simulink model "ECB"  (R2017a)
settings: Solver=ode4  StartTime=0.0  StopTime=1548.3  FixedStep=0.001  RelTol=1e-3  EnableMultiTasking=on
undefined symbols (not defined in the file or in its folder): magnitude, sgn, sigbuilder_block
libraries: simulink x1
(part 1 of 2)
settings Model: SimulationMode=accelerator  Creator=vepsalj1  LastModifiedBy=jariv
settings OptimizationCC: LifeSpan=inf  AccelVerboseBuild=on
settings DebuggingCC: AlgebraicLoopMsg=none  SFUnexpectedBacktrackingDiag=warning  SFNoUnconditionalDefaultTransitionDiag=warning  SFExecutionAtInitializationDiag=none
settings GRTTargetCC: TargetLangStandard=C89/C90 (ANSI)  GeneratePreprocessorConditionals=Disable all
settings ConfigComp: CovMetricSettings=dw  CovHtmlReporting=on  CovSaveCumulativeToWorkspaceVar=on  CovSaveSingleToWorkspaceVar=on  CovExternalEMLEnable=off

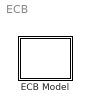
== system ECB ==
  ECB Model : Subsystem  mask{i=4.93, tRout=0.43, m=10500, Jm=0.63, Jt=8, head_wind=0, Cd=0.6, Ad=6.2, fr=0.008, kps=800, kis=0, kds=0, kps_park_multi=10, kpc=0.5, kic=80, kdc=0, Tmax=2080, Tbmax=30000, Rs=55e-3, Ls=5e-4, p=6, flux=0.42, Ppeak=207, Ich=282, Ids=395, soclim=90, vPart=4, aPart=4, x1=192, x2=2, Ah1=45, Rint1=2.5, C1=5, SOC0=85, Ta=20, Tb=20, Nnom=5000, NX=0, Rcor=1, Ccor=1, Ahcor=1, aux=5}
      mask prompts: i "Gear ratio (def 4.93)"; tRout "Tire diameter [m] (def 0.43)"; m "Vehicle mass [kg] (def 10500)"; Jm "Motor inertia [kgm2] (def 0.63)"; Jt "Tire inertia [kgm2] (def 8)"; head_wind "Head wind [m/s] (+ for drag)"; Cd "Coefficient of drag (def 0.493)"; Ad "Vehicle frontal area [m2] (def 6.2)"; fr "Rolling resistance coefficient (def 0.008)"; kps "Speed P gain (def  800)"; kis "Speed I gain (def 0)"; kds "Speed D gain (def 0)"; kps_park_multi "Speed P gain parking multiplier (def 10)"; kpc "Current P gain (def 0.5)"; kic "Current I gain (def 80)"; kdc "Current D gain (def 0)"; Tmax "Max. Motor Torque [Nm] (def 2080)"; Tbmax "Max. Braking Torque [Nm] (def 30 000)"; Rs "Internal resistance [ohm] (def 55e-3)"; Ls "Stator armature inductance [H] (def 5e-4)"; p "Number of pole pairs (def 6)"; flux "Flux induced by magnets [Vs] (def 0.42)"; Ppeak "Motor peak power (kW)"; Ich "Max. motor current when regenerating [A] (def 282)"; Ids "Max. motor current when motoring [A] (def 395)"; soclim "Battery SoC regeneration limit (%) (def 90)"; vPart "Regeneration velocity threshold [km/h] (def 4)"; aPart "Regeneration deceleration threshold [m/s^2] (def 4)"; x1 "Number of modules in series (def 192)"; x2 "Number of modules in parallel  (def 2)"; Ah1 "Nominal cell capacity [Ah] (def 45)"; Rint1 "Internal resistance of a module (mOhm) (@ 20 C) (def 2.5)"; C1 "Capacitance of a module [F] (def 5)"; SOC0 "State-of-Charge (%)"; Ta "Ambient temperature [C] (def 20)"; Tb "Battery temperature (C)"; Nnom "Number of cycles to 80 % aging (def 5000)"; NX "Cycle aging (20 % is EOL, 0 % is new)"; Rcor "Resistance gain"; Ccor "Capacitance gain"; Ahcor "Capacity gain"; aux "Aux power [kW] (constant) (def 5)"
      mask help:
      | Lithium-ion battery
      | - Max. Stepsize 0.2, otherwise there will be vibration in the beginning. Just to be on the safe side, recommended max.step 0.1
      mask init:
      | %MECHANICS
      | Jtot=(Jt*4)+(Jm*i^2);
      | %Four wheel plus the amplified inertia of the motor
      | 
      | %ELECTRONICS
      | PmotPeak=Ppeak*1000;
      | 
      | %BATTERY
      | SOD=[0;2.25000000000000;4;5.75000000000000;7.25000000000000;8.75000000000000;10.2500000000000;11.7500000000000;13.2500000000000;14.7500000000000;16.2500000000000;17.7500000000000;19.2500000000000;20.5000000000000;22;23.5000000000000;25;26.7500000000000;28.2500000000000;29.7500000000000;31.5000000000000;32.7500000000000;34.2500000000000;35.7500000000000;37.2500000000000;39.5000000000000;41.2500000000000;42.7500000000000;44.7500000000000;46.7500000000000;49;51;53.2500000000000;55.5000000000000;57.5000000000000;60;61.7500000000000;64;66.2500000000000;68.2500000000000;70.2500000000000;72.2500000000000;73.7500000000000;75.7500000000000;77.5000000000000;79;80.5000000000000;82;83.5000000000000;84.7500000000000;86.5000000000000;87.7500000000000;89.0000000000000;90.2500000000000;91.5000000000000;92.5000000000000;93.7500000000000;94.5000000000000;95;95.5000000000000;95.7500000000000;96.2500000000000;96.7500000000000;97.0000000000000;97.5000000000000;97.7500000000000;98.2500000000000;98.7500000000000;99.2500000000000;100];
      | VOLT=x1*1.015*[3.30000000000000;3.28450560652396;3.28018348623853;3.27431192660550;3.27308868501529;3.27125382262997;3.27003058103976;3.26819571865443;3.26697247706422;3.26574923547401;3.26452599388379;3.26269113149847;3.26146788990826;3.25963302752294;3.25779816513761;3.25596330275229;3.25474006116208;3.25290519877676;3.25107033639144;3.24862385321101;3.24678899082569;3.24495412844037;3.24311926605505;3.24128440366972;3.23944954128440;3.23761467889908;3.23516819571865;3.23272171253823;3.23027522935780;3.22844036697248;3.22599388379205;3.22354740061162;3.22110091743119;3.21865443425077;3.21559633027523;3.21253822629969;3.20948012232416;3.20703363914373;3.20458715596330;3.20214067278287;3.19969418960245;3.19663608562691;3.19296636085627;3.18868501529052;3.18379204892966;3.17828746177370;3.17278287461774;3.16666666666667;3.15932721712538;3.15076452599388;3.14097859327217;3.12996941896024;3.11712538226300;3.10305810397554;3.08654434250765;3.06880733944954;3.04740061162080;3.02354740061162;2.99785932721713;2.96850152905199;2.93486238532110;2.90061162079511;2.86330275229358;2.82354740061162;2.78012232415902;2.73425076452599;2.68409785932722;2.62782874617737;2.57033639143731;2.50305810397554];
      | 
      | VOLT0=interp1(SOD,VOLT,(1-SOC0/100));
      | % x1=number of cells in series
      | % x2=number of cells in parallel
      | 
      | Ah=x2*Ah1*Ahcor;
      | % Battery Characteristics
      | Qr=3600*Ah; %(coulomb) Nominal capacity in coulombs
      | 
      | N0=(Nnom/20)*NX; %From procentages of aging to number of cycles used
      | 
      | %R as a function of temperature, estimated from AMEsim battery (
      | %R = -0.000000063*Temp.^3+0.00000837*Temp.^2-0.000365*Temp+0.0068)
      | 
      | xx=(Rint1*10^-3)-(-0.000000063*20^3+0.00000837*20^2-0.000365*20);
      | Rint01 = -0.000000063*Tb^3+0.00000837*Tb^2-0.000365*Tb+xx;
      | 
      | Rint02=(x1/x2)*Rint01*Rcor;
      | R1=(2/3)*Rint02; %(ohm) (80 mOhm) (from Gao2002)
      | R2=(1/3)*Rint02; %(ohm) (40 mOhm)(from Gao2002)
      | 
      | Rint=(x1/x2)*Rint1*Rcor;
      | R1=(2/3)*Rint*10^-3; %(ohm) (80 mOhm) (from Gao2002)
      | R2=(1/3)*Rint*10^-3; %(ohm) (40 mOhm)(from Gao2002)
      | 
      | C=(x2/x1)*C1*Ccor;
      | 
      | %% Power converter efficiency
      | effeff=[0.148750893284055 0.459249842031262 0.572831006370283 0.661454547983232 0.702208498156483 0.745300650629634 0.774069453976362 0.802659853674854 0.819870547509622 0.839015378399121 0.851690885251339 0.864745206888717 0.872221885739442 0.879785746841656 0.890777178439945 0.900612362220784 0.905502967085794 0.910295193280307 0.914664248246699 0.916878485285563 0.919785184176078 0.917335161630957 0.920803182958674 0.925793859304388 0.930940164285346 0.936011371736695 0.937121595263058 0.938224789713163 0.941344451389100 0.942389340240952 0.941177012682751 0.942161786791917 0.946805761207415 0.951517305236046 0.956748293196982 0.957192859351870 0.957568033841468 0.956993932406603 0.960453080634668 0.958703134363870 0.958935623923192 0.960813757119483 0.960148641511847;0.382275397060378 0.606575062414118 0.724295084817057 0.763980132419977 0.817545815146612 0.836658234149830 0.850970215271699 0.875397571679227 0.885913726171233 0.897254928610336 0.906002057506642 0.916871389404069 0.925337547906322 0.929573292905226 0.935027508565980 0.934625050493851 0.936779709156045 0.942723985190616 0.945792130928845 0.947960897704374 0.947887831754402 0.950483214667466 0.954939155162541 0.957118148696677 0.962878037248519 0.964085567882039 0.964397321556185 0.966237886367941 0.967550686204577 0.967680328255962 0.968676606501984 0.968600791445791 0.969737387096799 0.970540279155023 0.970270355300112 0.969875112094269 0.970623441746216 0.971620597685068 0.971617448427293 0.973436842558703 0.971015950334548 0.972395281399074 0.972934205141957;0.502794468483159 0.704576784417921 0.780838362491516 0.824760271595067 0.855304468102641 0.874935150583253 0.890548161335983 0.898851103061955 0.911650918822123 0.920752385315524 0.923703036993863 0.938568143297259 0.941262344523035 0.939989162335414 0.947986636638787 0.950531267134112 0.950769184100132 0.953829085066537 0.957748210174090 0.952209232414559 0.959470289301486 0.965800711176068 0.969844708849249 0.970236996539206 0.971698393398446 0.973560393258196 0.972950737175279 0.973910716888667 0.975139162066989 0.975625795237705 0.974938242045002 0.974638822762701 0.975375940537886 0.975427862119037 0.975524897155774 0.977970674599018 0.977066843404792 0.976386481426328 0.978639106804244 0.976987258666757 0.976161252344463 0.974368520302056 0.979968848496111;0.590015102662206 0.757167014367670 0.802721182603195 0.855481189976114 0.875361411684403 0.886491064662271 0.907618702305879 0.917954995694953 0.926135352960324 0.929969047596192 0.934643440724457 0.946673327694363 0.949150648490242 0.952206770632412 0.953620700743328 0.958116293968123 0.960471764182804 0.960022428014383 0.964558913144813 0.964469991899858 0.967188838178770 0.973665568292064 0.973500122873302 0.975787459691329 0.976131734155535 0.975934048502296 0.977728917634797 0.975967753974241 0.977497590850481 0.976961490501139 0.976646573311052 0.976948671343312 0.977003373837591 0.977413505209625 0.977241769484167 0.978136863133043 0.983715860412863 0.972440548088471 0.976031098418230 0.976305098289204 0.983815037717926 0.990000000000000 0.980296964680289;0.642469564171041 0.782143695996117 0.834587558867662 0.867036501869607 0.885404521372931 0.900651198797785 0.918346940196575 0.926228607434163 0.933405508111231 0.940077144823606 0.941875513808993 0.949129235726833 0.955031705790567 0.955638703032255 0.959733157663852 0.961256947439685 0.964228704878266 0.965503729478674 0.967427866304563 0.970406018303361 0.975922234217047 0.976479479306018 0.977524713303582 0.978942094461665 0.977781595580544 0.977114802612142 0.975292354675851 0.977565938254442 0.977663963097884 0.970728918766358 0.978509263236759 0.979294318591674 0.978606184812507 0.980455355005113 0.977717973547513 0.977611212207795 0.977488362388515 0.983520834208511 0.978653676557568 0.977797224149179 0.976671295279777 0.982936790637227 0.974693280544320;0.666854189302077 0.796081554018545 0.853459995484673 0.875731344523075 0.894560218167283 0.910024324986280 0.920660243620183 0.936114908254807 0.937377010306665 0.943946530066235 0.947946898995783 0.955373031072732 0.956645495867027 0.961083778718095 0.961007216676884 0.965157442857362 0.965963755148971 0.968049149876401 0.971312101606815 0.975913333987052 0.975359086105523 0.977443627145109 0.977029983816712 0.978751343960785 0.978669311729546 0.980440204724162 0.984357530160600 0.978582708734772 0.979172562917930 0.978804034312948 0.978996524660769 0.978808094694211 0.978747993277991 0.978709803944595 0.984219208058756 0.978066410331978 0.977474370808590 0.976281712836119 0.976850901804032 0.970232997225184 0.990000000000000 0.990000000000000 0.990000000000000;0.693198974002651 0.812744420563275 0.861303411362365 0.888370040041046 0.899912367804584 0.912416422686382 0.927557031051808 0.934602759564506 0.939933212996785 0.947091254831535 0.951201311892576 0.959125411213696 0.959470857340005 0.961454980867527 0.963471596082249 0.965897069441330 0.967443349261464 0.968159753257309 0.972751289105061 0.976432852036816 0.977478975415255 0.978905952575006 0.978862035952765 0.979306529314671 0.979054079435176 0.979228864872502 0.980328291262954 0.979395165978778 0.979009717648825 0.979197157798663 0.979144584572849 0.979687221448110 0.979867607494733 0.978961695988816 0.982870884306758 0.976036523552125 0.970527543739429 0.990000000000000 0.990000000000000 0.990000000000000 0.990000000000000 0.990000000000000 0.990000000000000;0.723442421271799 0.819434992636961 0.866442600856177 0.887397491216575 0.912904261162542 0.915767451704052 0.930373806731795 0.937079106193214 0.942969048836058 0.948839064874878 0.953173425562567 0.957489332249449 0.963566641747761 0.964127874132415 0.964929847641875 0.966679582560640 0.968946853098627 0.970288863581759 0.975665835406012 0.977412335686879 0.979209315237733 0.978604269795064 0.979819900585854 0.979934412452209 0.980296834612691 0.979389810437186 0.979927925307359 0.979821966114863 0.980113197866812 0.978290737811240 0.978777326301659 0.978275795371243 0.977699190470578 0.976771188346836 0.990000000000000 0.990000000000000 0.990000000000000 0.990000000000000 0.990000000000000 0.990000000000000 0.990000000000000 0.990000000000000 0.990000000000000;0.748379721863994 0.841228290700447 0.864645554182945 0.893076811535185 0.909585899362390 0.920963299154172 0.934746905084107 0.941263940245672 0.943727860504373 0.950708651654628 0.954462263097205 0.960285791762753 0.962938135424456 0.963189598051574 0.965424092681620 0.967948124641425 0.968458535243243 0.974314778624769 0.976814364122101 0.979690184628213 0.979635217015122 0.979521508451437 0.979315060652411 0.980151729989435 0.979576323726992 0.979214145569015 0.980432559684310 0.979463877927784 0.978551029380815 0.978916907697418 0.978331589142382 0.978072711203139 0.990000000000000 0.990000000000000 0.990000000000000 0.990000000000000 0.990000000000000 0.990000000000000 0.990000000000000 0.990000000000000 0.990000000000000 0.990000000000000 0.990000000000000;0.739921993857994 0.842186224128038 0.872808349192410 0.897527110792011 0.911584252711211 0.926021034143323 0.931411696811273 0.943432421331771 0.946957435884837 0.952226260338947 0.955612156419591 0.961031292110199 0.963399102509892 0.965628015212985 0.967341907415101 0.968367188392990 0.970371532378770 0.975428592316753 0.978090341015957 0.978778385764394 0.979356164049638 0.979596787238044 0.979910905936328 0.980438856293780 0.979604150440873 0.979929471066156 0.978964026966460 0.979032120167408 0.978326079936520 0.976905872301957 0.990000000000000 0.990000000000000 0.990000000000000 0.990000000000000 0.990000000000000 0.990000000000000 0.990000000000000 0.990000000000000 0.990000000000000 0.990000000000000 0.990000000000000 0.990000000000000 0.990000000000000;0.764782550308260 0.845852311796918 0.877247852208968 0.900372955117317 0.916038722932507 0.928163498727814 0.936820012399945 0.945239540692551 0.949647219743305 0.952887074555875 0.956622739183461 0.961351963970377 0.965130871680347 0.966824861253174 0.967971837048059 0.969961656459446 0.972421208151907 0.977713476906919 0.978895920837105 0.979204761485868 0.979501173358470 0.979961739855176 0.979136090465072 0.979092361393791 0.979584768773003 0.979074142005905 0.978822659578355 0.977204544865391 0.976847711486498 0.969946121634669 0.990000000000000 0.990000000000000 0.990000000000000 0.990000000000000 0.990000000000000 0.990000000000000 0.990000000000000 0.990000000000000 0.990000000000000 0.990000000000000 0.990000000000000 0.990000000000000 0.990000000000000;0.781702272423770 0.850856501446949 0.887371611720997 0.903489514522146 0.917725906135129 0.930026206584236 0.940109652032560 0.944731124289788 0.950310533862187 0.953303758631013 0.956812198018296 0.962506374807609 0.964590641312338 0.966636502322765 0.968433304192319 0.970184913409236 0.976008771072597 0.978531617977455 0.978129704243536 0.981237408242478 0.978854028306741 0.979078648650488 0.978763489522089 0.978730864872159 0.977730529261954 0.977432502414182 0.977095679507429 0.990000000000000 0.976589342979380 0.990000000000000 0.990000000000000 0.990000000000000 0.990000000000000 0.990000000000000 0.990000000000000 0.990000000000000 0.990000000000000 0.990000000000000 0.990000000000000 0.990000000000000 0.990000000000000 0.990000000000000 0.990000000000000;0.781860601999475 0.858619139122591 0.886207437658841 0.909238965684978 0.919661646920446 0.932258700772937 0.938776654783832 0.945912837149306 0.950485214987112 0.953679120774217 0.957271780685473 0.962664754445029 0.965801175007356 0.967044978747895 0.969860460445190 0.971335906767362 0.977202313797035 0.978381886418063 0.979332030941349 0.979572138505992 0.977316490638900 0.979171153200939 0.978835122689707 0.978374231669299 0.977728938391822 0.976427492951010 0.975931850795350 0.990000000000000 0.990000000000000 0.990000000000000 0.990000000000000 0.990000000000000 0.990000000000000 0.990000000000000 0.990000000000000 0.990000000000000 0.990000000000000 0.990000000000000 0.990000000000000 0.990000000000000 0.990000000000000 0.990000000000000 0.990000000000000;0.806427770505860 0.855558035478508 0.888412877623268 0.908399525166180 0.922522501474443 0.935552000520952 0.940406178869038 0.947021368935208 0.949344944936003 0.954869173209383 0.959410423570906 0.963587411098435 0.966929808352867 0.967415809229096 0.968727991472268 0.970251786450644 0.977440666116929 0.978753821677089 0.978970693263824 0.978856971374949 0.978846286310281 0.978873792772526 0.978125058828133 0.978131119148409 0.990000000000000 0.990000000000000 0.990000000000000 0.990000000000000 0.990000000000000 0.990000000000000 0.990000000000000 0.990000000000000 0.990000000000000 0.990000000000000 0.990000000000000 0.990000000000000 0.990000000000000 0.990000000000000 0.990000000000000 0.990000000000000 0.990000000000000 0.990000000000000 0.990000000000000;0.802914656452277 0.866102036552135 0.891418534727099 0.911822813537450 0.923595507798633 0.934235480967195 0.940606934204237 0.947033096016217 0.951914879746563 0.956738225812308 0.958675347497316 0.963831456544986 0.966779657963926 0.969131103734101 0.969577178372756 0.973007968269652 0.977842057435959 0.978631185901036 0.979436274386932 0.978622168439258 0.979183621379517 0.978423428094268 0.977325150285219 0.990000000000000 0.990000000000000 0.990000000000000 0.990000000000000 0.990000000000000 0.990000000000000 0.990000000000000 0.990000000000000 0.990000000000000 0.990000000000000 0.990000000000000 0.990000000000000 0.990000000000000 0.990000000000000 0.990000000000000 0.990000000000000 0.990000000000000 0.990000000000000 0.990000000000000 0.990000000000000;0.806316271669901 0.866714464054199 0.889915902594281 0.913280217916478 0.920997404294818 0.932918677238818 0.941242245250447 0.947528694144073 0.952688936688243 0.955032171222350 0.959341430261600 0.963888452239613 0.965998412729959 0.968862420182887 0.969283164387637 0.973489743134963 0.979046417851264 0.979218461610945 0.978699032526251 0.979399408135760 0.978330920476013 0.973781382924854 0.990000000000000 0.990000000000000 0.990000000000000 0.990000000000000 0.990000000000000 0.990000000000000 0.990000000000000 0.990000000000000 0.990000000000000 0.990000000000000 0.990000000000000 0.990000000000000 0.990000000000000 0.990000000000000 0.990000000000000 0.990000000000000 0.990000000000000 0.990000000000000 0.990000000000000 0.990000000000000 0.990000000000000;0.818506587256520 0.869698259638791 0.894172011921041 0.912484031472958 0.927044868013181 0.935048577162901 0.941763150728836 0.946541040328738 0.952601726284618 0.956329267400120 0.959752567775117 0.964820724083667 0.967148536239869 0.968498944704594 0.969637351914519 0.974519925882493 0.978761034186936 0.977454398163469 0.979240976648830 0.978011719153542 0.978381072871212 0.990000000000000 0.990000000000000 0.990000000000000 0.990000000000000 0.990000000000000 0.990000000000000 0.990000000000000 0.990000000000000 0.990000000000000 0.990000000000000 0.990000000000000 0.990000000000000 0.990000000000000 0.990000000000000 0.990000000000000 0.990000000000000 0.990000000000000 0.990000000000000 0.990000000000000 0.990000000000000 0.990000000000000 0.990000000000000;0.827342304502606 0.874260028363306 0.898386130644280 0.916808038184915 0.924785053201677 0.937402027736400 0.941316240906288 0.948610444299530 0.952638876626130 0.957269227924557 0.958740932779589 0.964586476497988 0.966984968972377 0.967870675881160 0.969822561421690 0.974445100217118 0.978062839187441 0.979448786033379 0.978920230553390 0.990000000000000 0.990000000000000 0.990000000000000 0.990000000000000 0.990000000000000 0.990000000000000 0.990000000000000 0.990000000000000 0.990000000000000 0.990000000000000 0.990000000000000 0.990000000000000 0.990000000000000 0.990000000000000 0.990000000000000 0.990000000000000 0.990000000000000 0.990000000000000 0.990000000000000 0.990000000000000 0.990000000000000 0.990000000000000 0.990000000000000 0.990000000000000;0.828793161163873 0.883739270024190 0.897402900447648 0.920052572499606 0.925131871275858 0.936358309957953 0.941408397687570 0.947769074281290 0.953314327102907 0.958222584533746 0.960227033935968 0.964663888996119 0.965731980175840 0.968620781836763 0.971661231241175 0.976101555075591 0.978349022195705 0.979195957865253 0.990000000000000 0.990000000000000 0.990000000000000 0.990000000000000 0.990000000000000 0.990000000000000 0.990000000000000 0.990000000000000 0.990000000000000 0.990000000000000 0.990000000000000 0.990000000000000 0.990000000000000 0.990000000000000 0.990000000000000 0.990000000000000 0.990000000000000 0.990000000000000 0.990000000000000 0.990000000000000 0.990000000000000 0.990000000000000 0.990000000000000 0.990000000000000 0.990000000000000];
      | speedeff=[79.6471427140912 159.491674092761 239.794502112176 319.643916644608 399.467058331764 479.412025983156 559.645803766010 639.390275273601 719.340039720987 799.122962792120 879.087684356878 1039.17012652759 1119.03771579384 1198.84284647555 1279.14288147469 1358.95593436076 1438.90159841241 1518.73211278550 1598.58473667823 1678.84534292368 1758.69064040178 1838.41880868305 1918.39887551330 1998.56912352677 2078.51365890810 2158.43416550468 2238.12657870373 2318.03479953023 2398.30126442497 2478.22483680959 2558.03121244940 2637.95981477233 2718.12707868426 2797.86953270557 2877.85198791946 2957.69599779269 3037.71850367112 3117.85709273334 3197.61049277982 3277.76479518756 3357.12209861728 3428.99613524724 3511.61339840025];
      | torqueeff=[108.513506574596 214.974565339614 325.874686799886 435.179642275815 545.117342652292 655.382728555860 765.330817413053 874.387797583969 983.838250817781 1093.41246188526 1202.88111269057 1312.66815862822 1421.76834169744 1531.69740326202 1640.17226997275 1749.37273813806 1859.16221206858 1968.50220284129 2078.28136057567];
      mask DialogControl Control2 Prompt: The default values are based on Gao2002 paper about Dynamic Li-NMC batteries. Other sources have been used as well.

== system ECB/ECB Model ==
  Aux : Subsystem
  "Driver, Ctrl & Motor" : Subsystem
  Energy Storage : Subsystem
  Mechanics : Subsystem
  wires:
  Energy Storage/1(Ubat) -> "Driver, Ctrl & Motor"/1(Ubat), Aux/1(Ubat)
  Energy Storage/2(soc) -> "Driver, Ctrl & Motor"/2(soc)
  Mechanics/1(v) -> "Driver, Ctrl & Motor"/3(v)
  Mechanics/2(a) -> "Driver, Ctrl & Motor"/4(a)
  "Driver, Ctrl & Motor"/2(Tx) -> Mechanics/1(Tx)
  "Driver, Ctrl & Motor"/1(ia) -> Energy Storage/2(iM)
  Aux/1(iAux) -> Energy Storage/1(iAux)

== system ECB/ECB Model/Aux ==
  Ubat : Inport
  AUX [kW to W] : Constant  Value=aux*1000
  Add : Sum
  Ambient Temp : Constant  Value=Ta
  AuxTot : Subsystem  Tag=STV Subsys  Commented=on  LoadFcn=sigbuilder_block('load');  StartFcn=sigbuilder_block('start');  StopFcn=sigbuilder_block('stop');  ClipboardFcn=sigbuilder_block('clipboard');  mask(Sigbuilder block){tuvar=[0:10]}
      mask help: Simulink:masks:SigbuilderBlock_MD
      mask init:
      | if ~strcmp(get_param(bdroot(gcbh),'SimulationStatus'),'stopped') tuvar = sigbuilder_block('maskInit'); end
      settings: CopyFcn=sigbuilder_block('copy');  DeleteFcn=sigbuilder_block('delete');  ModelCloseFcn=sigbuilder_block('modelClose');  PreSaveFcn=sigbuilder_block('preSave');  PauseFcn=sigbuilder_block('pause');  ContinueFcn=sigbuilder_block('continue');  NameChangeFcn=sigbuilder_block('namechange');  OpenFcn=sigbuilder_block('open',[6 30 1428 682.5 ]);  CloseFcn=sigbuilder_block('close');
      mask Display: plot(0, 0, 100, 100,[2, 2, 32, 32, 2], [68, 8, 8, 68, 68],[32, 2], [38, 38], [32, 19, 2],[53, 60, 44], [32, 17, 17, 2],[16, 16, 31, 31]);txt = getActiveGroup(gcbh);text(2, 100, txt,'verticalAlignment', 'top');
  Gain : Gain  Commented=on  Gain=1000
  HVAC Power : Lookup_n-D  NumberOfTableDimensions=1  BreakpointsForDimension1=|  Table=|  InternalRulePriority=Speed  RndMeth=Simplest  InputSameDT=on
      BreakpointsForDimension1=|
      | [-30.0000
      |   -27.7680
      |   -25.6721
      |   -23.1831
      |   -19.9733
      |   -16.6978
      |   -13.8805
      |   -12.7007
      |   -10.7343
      |    -8.9644
      |    -7.1281
      |    -5.4232
      |    -3.1932
      |    -1.4876
      |     0.8084
      |     2.7110
      |     5.2042
      |     7.5666
      |    10.6510
      |    13.2108
      |    14.7861
      |    16.5593
      |    18.6610
      |    20.5663
      |    22.1443
      |    23.9195
      |    25.1692
      |    26.4203
      |    27.8030
      |    28.7907
      |    29.5812
      |    30.0418]
      Table=|
      | [22.3000
      |    20.0013
      |    18.1962
      |    16.1024
      |    13.5031
      |    10.9040
      |     8.8464
      |     8.1607
      |     7.0058
      |     6.0676
      |     5.3823
      |     4.6608
      |     3.9396
      |     3.4709
      |     2.8581
      |     2.4258
      |     1.9215
      |     1.5978
      |     1.2383
      |     1.0954
      |     1.0241
      |     1.3503
      |     1.7490
      |     2.3281
      |     3.3045
      |     4.3533
      |     5.2572
      |     6.7392
      |     8.2935
      |     9.4501
      |    10.4983
      |    10.9321]*1000
  I=P/U : Product  Inputs=*/
  Saturation : Saturate  UpperLimit=5000  LowerLimit=300
  iAux : Outport
  wires:
  I=P/U/1 -> iAux/1
  Ubat/1 -> Saturation/1
  Ambient Temp/1 -> HVAC Power/1
  Saturation/1 -> I=P/U/2
  AuxTot/1(vel) -> Gain/1
  AUX [kW to W]/1 -> Add/1
  HVAC Power/1 -> Add/2
  Add/1 -> I=P/U/1

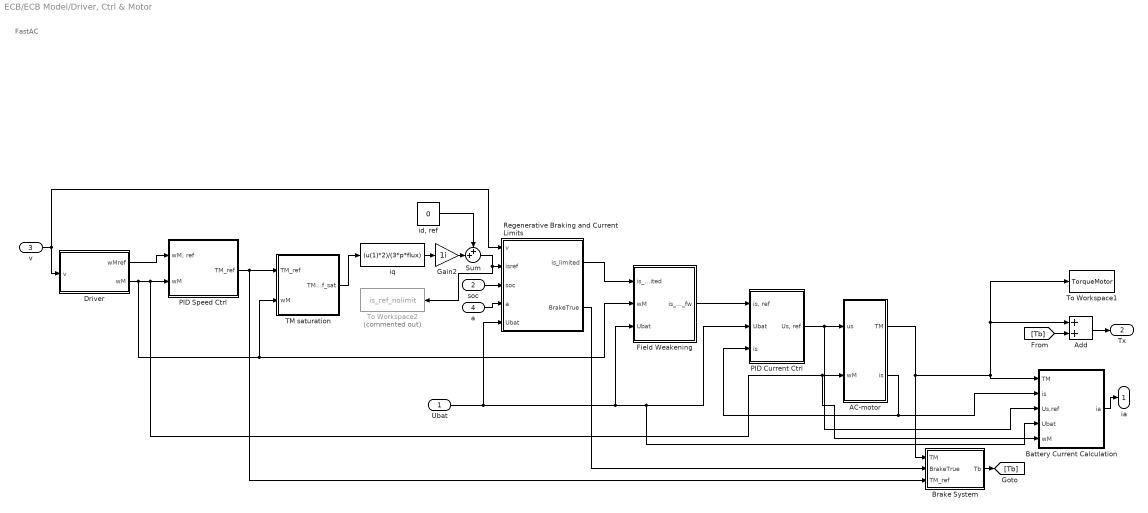
== system ECB/ECB Model/Driver, Ctrl & Motor ==
  note: FastAC
  Ubat : Inport
  soc : Inport  Port=2
  v : Inport  Port=3
  a : Inport  Port=4
  AC-motor : Subsystem
  Add : Sum
  Battery Current Calculation : Subsystem
  Brake System : Subsystem
  Driver : Subsystem
  Field Weakening : Subsystem
  Gain2 : Gain  Gain=1i
  PID Current Ctrl : Subsystem
  PID Speed Ctrl : Subsystem
  Regenerative Braking and Current Limits : Subsystem
  Sum : Sum  Inputs=++|
  TM saturation : Subsystem
  To Workspace1 : ToWorkspace  VariableName=TorqueMotor  SampleTime=-1
      settings: Save2DSignal=2-D array (concatenate along first dimension)
  To Workspace2 : ToWorkspace  Commented=on  VariableName=is_ref_nolimit  SampleTime=-1
      settings: Save2DSignal=2-D array (concatenate along first dimension)
  "id, ref" : Constant  Value=0
  iq : Fcn  Expr=(u(1)*2)/(3*p*flux)
  ia : Outport
  Tx : Outport  Port=2
  wires:
  Battery Current Calculation/1(ia) -> ia/1
  soc/1 -> Regenerative Braking and Current Limits/3(soc)
  v/1 -> Driver/1(v), Regenerative Braking and Current Limits/1(v)
  a/1 -> Regenerative Braking and Current Limits/4(a)
  Ubat/1 -> Regenerative Braking and Current Limits/5(Ubat), Field Weakening/3(Ubat), Battery Current Calculation/4(Ubat), PID Current Ctrl/2(Ubat)
  PID Speed Ctrl/1(TM_ref) -> TM saturation/1(TM_ref), Brake System/3(TM_ref)
  "id, ref"/1 -> Sum/1
  PID Current Ctrl/1("Us, ref") -> AC-motor/1(us), Battery Current Calculation/3(Us,ref)
  Driver/2(wM) -> PID Speed Ctrl/2(wM), Battery Current Calculation/5(wM), AC-motor/2(wM), TM saturation/2(wM), Field Weakening/2(wM)
  Gain2/1 -> Sum/2
  AC-motor/2(is) -> PID Current Ctrl/3(is), Battery Current Calculation/2(is)
  Driver/1(wMref) -> PID Speed Ctrl/1("wM, ref")
  Add/1 -> Tx/1
  [Tb] -> Add/2
  Brake System/1(Tb) -> [Tb]
  Sum/1 -> To Workspace2/1, Regenerative Braking and Current Limits/2(isref)
  iq/1 -> Gain2/1
  Regenerative Braking and Current Limits/2(BrakeTrue) -> Brake System/2(BrakeTrue)
  AC-motor/1(TM) -> To Workspace1/1, Add/1, Battery Current Calculation/1(TM), Brake System/1(TM)
  Field Weakening/1(is_ref_fw) -> PID Current Ctrl/1("is, ref")
  Regenerative Braking and Current Limits/1(is_limited) -> Field Weakening/1(is_limited)
  TM saturation/1(TMref_sat) -> iq/1

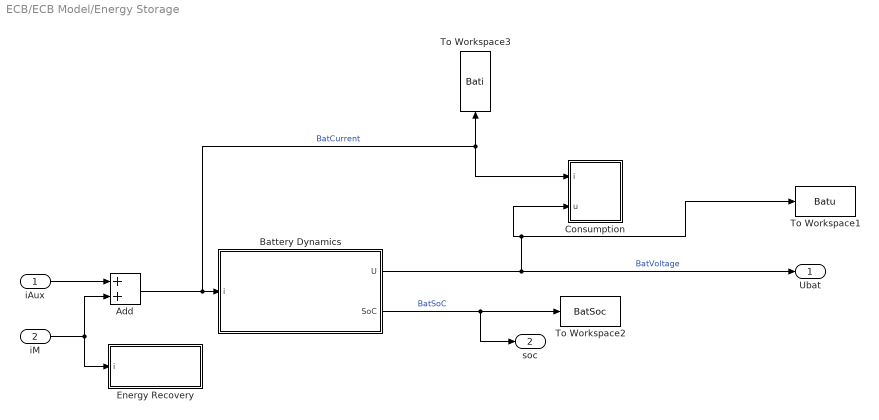
== system ECB/ECB Model/Energy Storage ==
  iAux : Inport
  iM : Inport  Port=2
  Add : Sum
  Battery Dynamics : Subsystem
  Consumption : Subsystem
  Energy Recovery : Subsystem
  To Workspace1 : ToWorkspace  VariableName=Batu  SampleTime=-1
  To Workspace2 : ToWorkspace  VariableName=BatSoc  SampleTime=-1
  To Workspace3 : ToWorkspace  VariableName=Bati  SampleTime=-1
  Ubat : Outport
  soc : Outport  Port=2
  wires:
  iAux/1 -> Add/1
  iM/1 -> Add/2, Energy Recovery/1(i)
  Add/1 -> To Workspace3/1, Consumption/1(i), Battery Dynamics/1(i)  "BatCurrent"
  Battery Dynamics/1(U) -> Consumption/2(u), To Workspace1/1, Ubat/1  "BatVoltage"
  Battery Dynamics/2(SoC) -> To Workspace2/1, soc/1  "BatSoC"

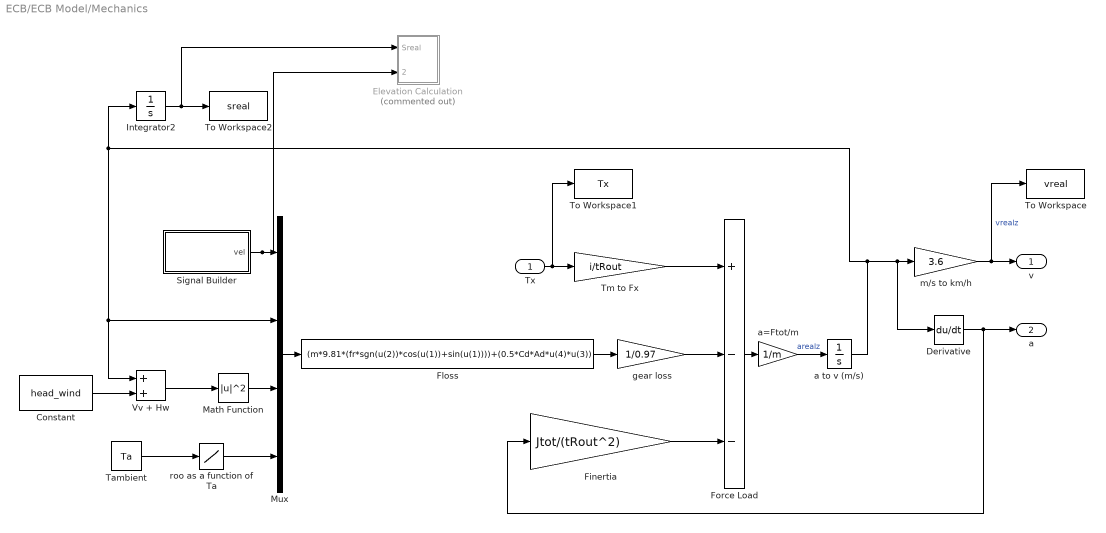
== system ECB/ECB Model/Mechanics ==
  Tx : Inport
  Constant : Constant  Value=head_wind
  Derivative : Derivative
  Elevation Calculation : Subsystem  Commented=on
  Finertia : Gain  Gain=Jtot/(tRout^2)
  Floss : Fcn  Expr=(m*9.81*(fr*sgn(u(2))*cos(u(1))+sin(u(1))))+(0.5*Cd*Ad*u(4)*u(3))
  Force Load : Sum  Inputs=+--
  Integrator2 : Integrator
  Math Function : Math  Operator=magnitude^2  SaturateOnIntegerOverflow=on
  Mux : Mux
  Signal Builder : Subsystem  Tag=STV Subsys  LoadFcn=sigbuilder_block('load');  StartFcn=sigbuilder_block('start');  StopFcn=sigbuilder_block('stop');  ClipboardFcn=sigbuilder_block('clipboard');  mask(Sigbuilder block){tuvar=[0:10]}
      mask help: Simulink:masks:SigbuilderBlock_MD
      mask init:
      | if ~strcmp(get_param(bdroot(gcbh),'SimulationStatus'),'stopped') tuvar = sigbuilder_block('maskInit'); end
      settings: CopyFcn=sigbuilder_block('copy');  DeleteFcn=sigbuilder_block('delete');  ModelCloseFcn=sigbuilder_block('modelClose');  PreSaveFcn=sigbuilder_block('preSave');  PauseFcn=sigbuilder_block('pause');  ContinueFcn=sigbuilder_block('continue');  NameChangeFcn=sigbuilder_block('namechange');  OpenFcn=sigbuilder_block('open',[0 30 1440 723 ]);  CloseFcn=sigbuilder_block('close');
      mask Display: plot(0, 0, 100, 100,[2, 2, 32, 32, 2], [68, 8, 8, 68, 68],[32, 2], [38, 38], [32, 19, 2],[53, 60, 44], [32, 17, 17, 2],[16, 16, 31, 31]);txt = getActiveGroup(gcbh);text(2, 100, txt,'verticalAlignment', 'top');
  Tambient : Constant  Value=Ta
  Tm to Fx : Gain  Gain=i/tRout
  To Workspace : ToWorkspace  VariableName=vreal  SampleTime=-1
      settings: Save2DSignal=2-D array (concatenate along first dimension)
  To Workspace1 : ToWorkspace  VariableName=Tx  SampleTime=-1
      settings: Save2DSignal=2-D array (concatenate along first dimension)
  To Workspace2 : ToWorkspace  VariableName=sreal  SampleTime=-1
      settings: Save2DSignal=2-D array (concatenate along first dimension)
  Vv + Hw : Sum
  a to v (m/s) : Integrator  LimitOutput=on  UpperSaturationLimit=100  LowerSaturationLimit=0
  a=Ftot/m : Gain  Gain=1/m
  gear loss : Gain  Gain=1/0.97
  m/s to km/h : Gain  Gain=3.6
  roo as a function of Ta : Lookup_n-D  NumberOfTableDimensions=1  BreakpointsForDimension1="[-25   -20   -15   -10    -5     0     5    10    15    20    25    30    35]"  Table="[ 1.4224    1.3943    1.3673    1.3413    1.3163    1.2922    1.2690    1.2466    1.2250    1.2041    1.1839    1.1644   1.1455]"  InternalRulePriority=Speed  RndMeth=Simplest  InputSameDT=on
  v : Outport
  a : Outport  Port=2
  wires:
  Tx/1 -> To Workspace1/1, Tm to Fx/1
  Tm to Fx/1 -> Force Load/1
  Tambient/1 -> roo as a function of Ta/1
  Mux/1 -> Floss/1
  Math Function/1 -> Mux/3
  roo as a function of Ta/1 -> Mux/4
  Constant/1 -> Vv + Hw/2
  Vv + Hw/1 -> Math Function/1
  a to v (m/s)/1 -> Derivative/1, m/s to km/h/1, Integrator2/1, Vv + Hw/1, Mux/2
  m/s to km/h/1 -> v/1, To Workspace/1  "vrealz"
  Force Load/1 -> a=Ftot/m/1
  a=Ftot/m/1 -> a to v (m/s)/1  "arealz"
  Derivative/1 -> Finertia/1, a/1
  Signal Builder/1(vel) -> Elevation Calculation/2(Grade), Mux/1
  Finertia/1 -> Force Load/3
  Floss/1 -> gear loss/1
  Integrator2/1 -> Elevation Calculation/1(Sreal), To Workspace2/1
  gear loss/1 -> Force Load/2

== system ECB/ECB Model/Aux/AuxTot ==
  Demux : Demux  Tag=STV Demux  Outputs=1
  FromWs : FromWorkspace  Tag=STV FromWs  VariableName=tuvar  SampleTime=0
      SigBuilderData=|
      | common.afterFinalStr = 'Extrapolate'
      | common.sampleTime = 0
      | dataSet(1).timeRange = [0 10]
      | dataSet(1).name = 'Group 1'
      | dataSet(2).timeRange = [0 1567.5]
      | dataSet(2).name = 'AuxTotKw'
      | sbobj.Groups(1).Name = 'Group 1'
      | sbobj.Groups(1).Signals.Name = 'vel'
      | sbobj.Groups(1).Signals.XData = [0 4 4 6 6 10]
      | sbobj.Groups(1).Signals.YData = [0 0 1 1 0 0]
      | sbobj.Groups(2).Name = 'AuxTotKw'
      | sbobj.Groups(2).Signals.Name = 'vel'
      | sbobj.Groups(2).Signals.XData = [0 0.1 0.2 0.3 0.4 0.5 0.6 0.7 0.8 0.9 1 1.1 ... (15676 elements, 1x15676)]
      | sbobj.Groups(2).Signals.YData = [2.71091459439 2.86329264392 3.01068577674 3.15470865145 3.29659201305 3.43712426111 3.57649187195 3.71394032146 3.8469766966 3.96893960152 4.06210025267 4.09001640206 ... (15676 elements, 1x15676)]
      | sbobj.Groups(2).TimeRange = [0 1567.5]
  vel : Outport  Tag=STV Outport
  wires:
  Demux/1 -> vel/1
  FromWs/1 -> Demux/1

== system ECB/ECB Model/Driver, Ctrl & Motor/AC-motor ==
  us : Inport
  wM : Inport  Port=2
  Electromagnetic Torque : Subsystem
  Flux Equations : Subsystem
  To Workspace1 : ToWorkspace  Commented=on  VariableName=is_complex  SampleTime=-1
  To Workspace2 : ToWorkspace  Commented=on  VariableName=psis_complex  SampleTime=-1
  Voltage Equations : Subsystem
  TM : Outport
  is : Outport  Port=2
  wires:
  Voltage Equations/1(psis) -> To Workspace2/1, Electromagnetic Torque/2(psis), Flux Equations/1(psis)
  Flux Equations/1(is) -> is/1, Electromagnetic Torque/1(is), Voltage Equations/2(is), To Workspace1/1
  us/1 -> Voltage Equations/1(us)
  wM/1 -> Voltage Equations/3(wM)
  Electromagnetic Torque/1(TM) -> TM/1

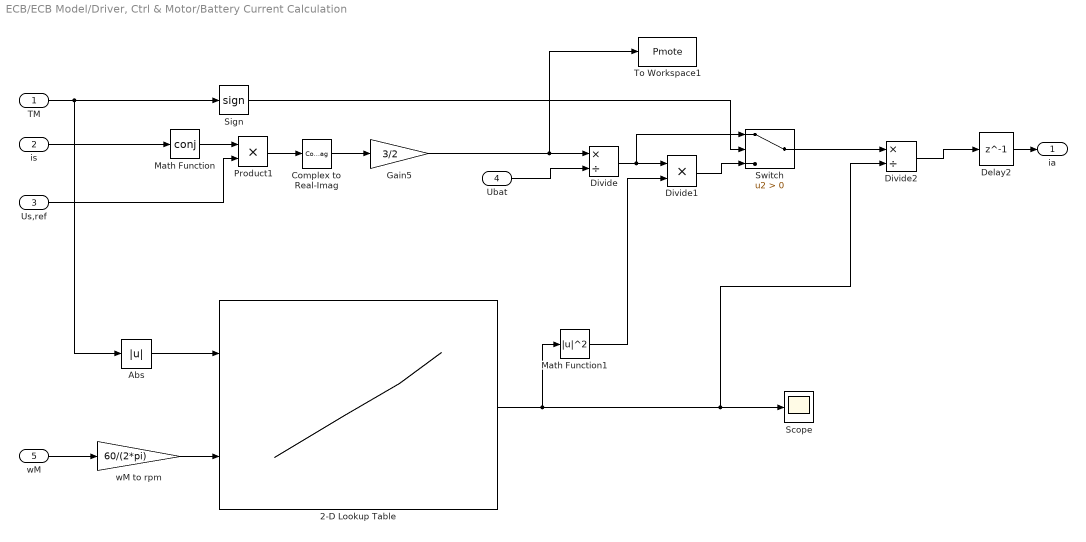
== system ECB/ECB Model/Driver, Ctrl & Motor/Battery Current Calculation ==
  TM : Inport
  is : Inport  Port=2
  Us,ref : Inport  Port=3
  Ubat : Inport  Port=4
  wM : Inport  Port=5
  2-D Lookup Table : Lookup_n-D  BreakpointsForDimension1=torqueeff  BreakpointsForDimension2=speedeff  Table=effeff  ExtrapMethod=Clip  UseLastTableValue=on  InternalRulePriority=Speed  RndMeth=Simplest  InputSameDT=on
  Abs : Abs
  Complex to Real-Imag : ComplexToRealImag  Output=Real
  Delay2 : Delay  DelayLength=1  InitialCondition=0
  Divide : Product  Inputs=*/
  Divide1 : Product  Inputs=**
  Divide2 : Product  Inputs=*/
  Gain5 : Gain  Gain=3/2
  Math Function : Math  Operator=conj  SaturateOnIntegerOverflow=on
  Math Function1 : Math  Operator=magnitude^2  SaturateOnIntegerOverflow=on
  Product1 : Product
  Scope : Scope
  Sign : Signum
  Switch : Switch  Criteria=u2 > Threshold
  To Workspace1 : ToWorkspace  VariableName=Pmote  SampleTime=-1
      settings: Save2DSignal=2-D array (concatenate along first dimension)
  wM to rpm : Gain  Gain=60/(2*pi)
  ia : Outport
  wires:
  Sign/1 -> Switch/2
  Switch/1 -> Divide2/1
  Divide1/1 -> Switch/3
  TM/1 -> Sign/1, Abs/1
  Divide/1 -> Divide1/1, Switch/1
  Product1/1 -> Complex to Real-Imag/1
  Complex to Real-Imag/1 -> Gain5/1
  Math Function/1 -> Product1/1
  Ubat/1 -> Divide/2
  Us,ref/1 -> Product1/2
  Delay2/1 -> ia/1
  Divide2/1 -> Delay2/1
  Gain5/1 -> To Workspace1/1, Divide/1
  is/1 -> Math Function/1
  wM/1 -> wM to rpm/1
  wM to rpm/1 -> 2-D Lookup Table/2
  Abs/1 -> 2-D Lookup Table/1
  2-D Lookup Table/1 -> Divide2/2, Scope/1, Math Function1/1
  Math Function1/1 -> Divide1/2

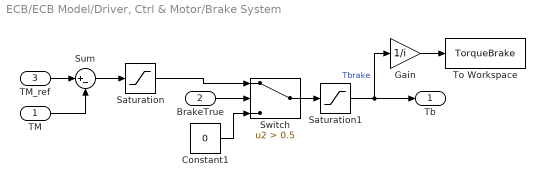
== system ECB/ECB Model/Driver, Ctrl & Motor/Brake System ==
  TM : Inport
  BrakeTrue : Inport  Port=2
  TM_ref : Inport  Port=3
  Constant1 : Constant  Value=0
  Gain : Gain  Gain=1/i
  Saturation : Saturate  UpperLimit=0  LowerLimit=-Tbmax/i
  Saturation1 : Saturate  UpperLimit=0  LowerLimit=-Tbmax/i
  Sum : Sum  Inputs=|+-
  Switch : Switch  Criteria=u2 > Threshold  Threshold=0.5
  To Workspace : ToWorkspace  VariableName=TorqueBrake  SampleTime=-1
  Tb : Outport
  wires:
  Saturation1/1 -> Gain/1, Tb/1  "Tbrake"
  Constant1/1 -> Switch/3
  Switch/1 -> Saturation1/1
  BrakeTrue/1 -> Switch/2
  TM/1 -> Sum/2
  TM_ref/1 -> Sum/1
  Sum/1 -> Saturation/1
  Saturation/1 -> Switch/1
  Gain/1 -> To Workspace/1

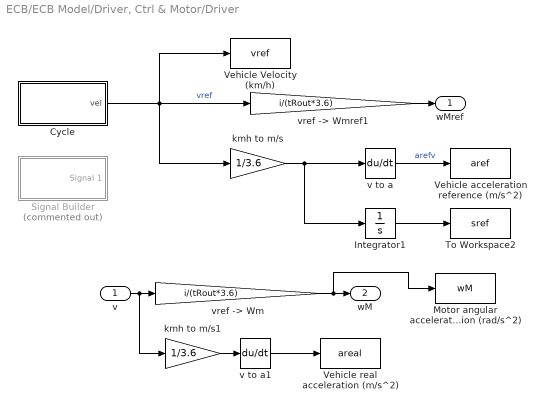
== system ECB/ECB Model/Driver, Ctrl & Motor/Driver ==
  v : Inport
  Cycle : Subsystem  Tag=STV Subsys  LoadFcn=sigbuilder_block('load');  StartFcn=sigbuilder_block('start');  StopFcn=sigbuilder_block('stop');  ClipboardFcn=sigbuilder_block('clipboard');  mask(Sigbuilder block){tuvar=[0:10]}
      mask help: Simulink:masks:SigbuilderBlock_MD
      mask init:
      | if ~strcmp(get_param(bdroot(gcbh),'SimulationStatus'),'stopped') tuvar = sigbuilder_block('maskInit'); end
      settings: CopyFcn=sigbuilder_block('copy');  DeleteFcn=sigbuilder_block('delete');  ModelCloseFcn=sigbuilder_block('modelClose');  PreSaveFcn=sigbuilder_block('preSave');  PauseFcn=sigbuilder_block('pause');  ContinueFcn=sigbuilder_block('continue');  NameChangeFcn=sigbuilder_block('namechange');  OpenFcn=sigbuilder_block('open',[6 30 1428 682.5 ]);  CloseFcn=sigbuilder_block('close');
      mask Display: plot(0, 0, 100, 100,[2, 2, 32, 32, 2], [68, 8, 8, 68, 68],[32, 2], [38, 38], [32, 19, 2],[53, 60, 44], [32, 17, 17, 2],[16, 16, 31, 31]);txt = getActiveGroup(gcbh);text(2, 100, txt,'verticalAlignment', 'top');
  Integrator1 : Integrator
  Motor angular acceleration (rad/s^2) : ToWorkspace  VariableName=wM  SampleTime=-1
      settings: Save2DSignal=2-D array (concatenate along first dimension)
  Signal Builder : Subsystem  Tag=STV Subsys  Commented=on  LoadFcn=sigbuilder_block('load');  StartFcn=sigbuilder_block('start');  StopFcn=sigbuilder_block('stop');  ClipboardFcn=sigbuilder_block('clipboard');  mask(Sigbuilder block){tuvar=[0:10]}
      mask help: Simulink:masks:SigbuilderBlock_MD
      mask init:
      | if ~strcmp(get_param(bdroot(gcbh),'SimulationStatus'),'stopped') tuvar = sigbuilder_block('maskInit'); end
      settings: CopyFcn=sigbuilder_block('copy');  DeleteFcn=sigbuilder_block('delete');  ModelCloseFcn=sigbuilder_block('modelClose');  PreSaveFcn=sigbuilder_block('preSave');  PauseFcn=sigbuilder_block('pause');  ContinueFcn=sigbuilder_block('continue');  NameChangeFcn=sigbuilder_block('namechange');  OpenFcn=sigbuilder_block('open',[6 30 1428 682.5 ]);  CloseFcn=sigbuilder_block('close');
      mask Display: plot(0, 0, 100, 100,[2, 2, 32, 32, 2], [68, 8, 8, 68, 68],[32, 2], [38, 38], [32, 19, 2],[53, 60, 44], [32, 17, 17, 2],[16, 16, 31, 31]);txt = getActiveGroup(gcbh);text(2, 100, txt,'verticalAlignment', 'top');
  To Workspace2 : ToWorkspace  VariableName=sref  SampleTime=-1
      settings: Save2DSignal=2-D array (concatenate along first dimension)
  Vehicle Velocity (km/h) : ToWorkspace  VariableName=vref  SampleTime=-1
      settings: Save2DSignal=2-D array (concatenate along first dimension)
  Vehicle acceleration reference (m/s^2) : ToWorkspace  VariableName=aref  SampleTime=-1
      settings: Save2DSignal=2-D array (concatenate along first dimension)
  Vehicle real acceleration (m/s^2) : ToWorkspace  VariableName=areal  SampleTime=-1
      settings: Save2DSignal=2-D array (concatenate along first dimension)
  kmh to m/s : Gain  Gain=1/3.6
  kmh to m/s1 : Gain  Gain=1/3.6
  v to a : Derivative
  v to a1 : Derivative
  "vref -> Wm" : Gain  Gain=i/(tRout*3.6)
  "vref -> Wmref1" : Gain  Gain=i/(tRout*3.6)
  wMref : Outport
  wM : Outport  Port=2
  wires:
  "vref -> Wmref1"/1 -> wMref/1
  kmh to m/s/1 -> Integrator1/1, v to a/1
  v to a/1 -> Vehicle acceleration reference (m/s^2)/1  "arefv"
  v/1 -> kmh to m/s1/1, "vref -> Wm"/1
  Integrator1/1 -> To Workspace2/1
  kmh to m/s1/1 -> v to a1/1
  v to a1/1 -> Vehicle real acceleration (m/s^2)/1
  "vref -> Wm"/1 -> Motor angular acceleration (rad/s^2)/1, wM/1
  Cycle/1(vel) -> kmh to m/s/1, "vref -> Wmref1"/1, Vehicle Velocity (km/h)/1  "vref"

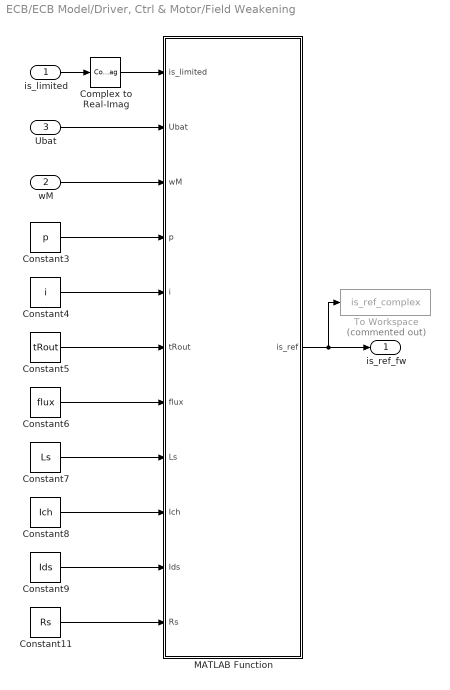
== system ECB/ECB Model/Driver, Ctrl & Motor/Field Weakening ==
  is_limited : Inport
  wM : Inport  Port=2
  Ubat : Inport  Port=3
  Complex to Real-Imag : ComplexToRealImag  Output=Imag
  Constant11 : Constant  Value=Rs
  Constant3 : Constant  Value=p
  Constant4 : Constant  Value=i
  Constant5 : Constant  Value=tRout
  Constant6 : Constant  Value=flux
  Constant7 : Constant  Value=Ls
  Constant8 : Constant  Value=Ich
  Constant9 : Constant  Value=Ids
  MATLAB Function : MATLAB Function  TreatAsAtomicUnit=on
  To Workspace : ToWorkspace  Commented=on  VariableName=is_ref_complex  SampleTime=-1
  is_ref_fw : Outport
  wires:
  is_limited/1 -> Complex to Real-Imag/1
  Constant3/1 -> MATLAB Function/4(p)
  Constant4/1 -> MATLAB Function/5(i)
  Constant5/1 -> MATLAB Function/6(tRout)
  Constant7/1 -> MATLAB Function/8(Ls)
  Constant6/1 -> MATLAB Function/7(flux)
  MATLAB Function/1(is_ref) -> To Workspace/1, is_ref_fw/1
  Complex to Real-Imag/1 -> MATLAB Function/1(is_limited)
  wM/1 -> MATLAB Function/3(wM)
  Ubat/1 -> MATLAB Function/2(Ubat)
  Constant9/1 -> MATLAB Function/10(Ids)
  Constant8/1 -> MATLAB Function/9(Ich)
  Constant11/1 -> MATLAB Function/11(Rs)

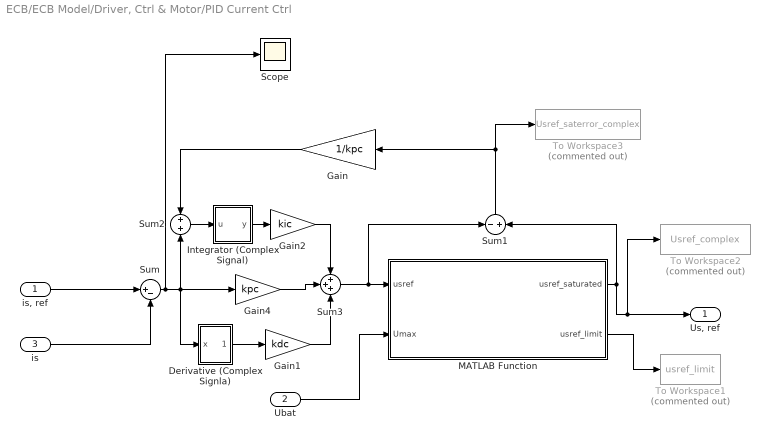
== system ECB/ECB Model/Driver, Ctrl & Motor/PID Current Ctrl ==
  "is, ref" : Inport
  Ubat : Inport  Port=2
  is : Inport  Port=3
  Derivative (Complex Signla) : Subsystem
  Gain : Gain  Gain=1/kpc
  Gain1 : Gain  Gain=kdc
  Gain2 : Gain  Gain=kic
  Gain4 : Gain  Gain=kpc
  Integrator (Complex Signal) : Subsystem
      mask Display: disp('1/s');
  MATLAB Function : MATLAB Function  TreatAsAtomicUnit=on
  Scope : Scope
  Sum : Sum  Inputs=|+-
  Sum1 : Sum  Inputs=-+
  Sum2 : Sum
  Sum3 : Sum  Inputs=+++
  To Workspace1 : ToWorkspace  Commented=on  VariableName=usref_limit  SampleTime=-1
  To Workspace2 : ToWorkspace  Commented=on  VariableName=Usref_complex  SampleTime=-1
  To Workspace3 : ToWorkspace  Commented=on  VariableName=Usref_saterror_complex  SampleTime=-1
  "Us, ref" : Outport
  wires:
  Sum1/1 -> To Workspace3/1, Gain/1
  Gain/1 -> Sum2/1
  Sum2/1 -> Integrator (Complex Signal)/1(u)
  Ubat/1 -> MATLAB Function/2(Umax)
  Sum3/1 -> MATLAB Function/1(usref), Sum1/1
  Gain2/1 -> Sum3/1
  Gain4/1 -> Sum3/2
  Integrator (Complex Signal)/1(y) -> Gain2/1
  Sum/1 -> Scope/1, Derivative (Complex Signla)/1(x), Gain4/1, Sum2/2
  Gain1/1 -> Sum3/3
  Derivative (Complex Signla)/1(dx) -> Gain1/1
  MATLAB Function/2(usref_limit) -> To Workspace1/1
  "is, ref"/1 -> Sum/1
  is/1 -> Sum/2
  MATLAB Function/1(usref_saturated) -> "Us, ref"/1, To Workspace2/1, Sum1/2

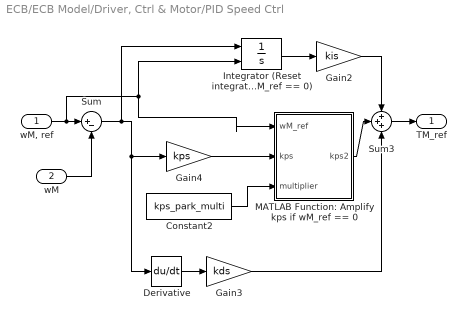
== system ECB/ECB Model/Driver, Ctrl & Motor/PID Speed Ctrl ==
  "wM, ref" : Inport
  wM : Inport  Port=2
  Constant2 : Constant  Value=kps_park_multi
  Derivative : Derivative
  Gain2 : Gain  Gain=kis
  Gain3 : Gain  Gain=kds
  Gain4 : Gain  Gain=kps
  Integrator (Reset integrator if wM_ref == 0) : Integrator  ExternalReset=falling
  MATLAB Function: Amplify kps if wM_ref == 0 : MATLAB Function  TreatAsAtomicUnit=on
  Sum : Sum  Inputs=|+-
  Sum3 : Sum  Inputs=+++
  TM_ref : Outport
  wires:
  Sum/1 -> Integrator (Reset integrator if wM_ref == 0)/1, Derivative/1, Gain4/1
  Integrator (Reset integrator if wM_ref == 0)/1 -> Gain2/1
  Gain2/1 -> Sum3/1
  wM/1 -> Sum/2
  Gain3/1 -> Sum3/3
  Derivative/1 -> Gain3/1
  "wM, ref"/1 -> MATLAB Function: Amplify kps if wM_ref == 0/1(wM_ref), Integrator (Reset integrator if wM_ref == 0)/2, Sum/1
  Gain4/1 -> MATLAB Function: Amplify kps if wM_ref == 0/2(kps)
  MATLAB Function: Amplify kps if wM_ref == 0/1(kps2) -> Sum3/2
  Sum3/1 -> TM_ref/1
  Constant2/1 -> MATLAB Function: Amplify kps if wM_ref == 0/3(multiplier)

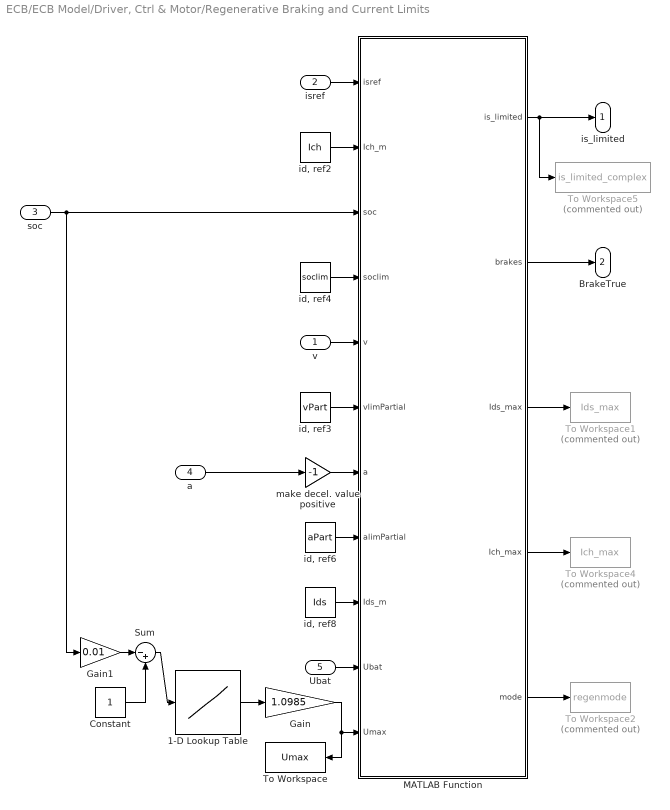
== system ECB/ECB Model/Driver, Ctrl & Motor/Regenerative Braking and Current Limits ==
  v : Inport
  isref : Inport  Port=2
  soc : Inport  Port=3
  a : Inport  Port=4
  Ubat : Inport  Port=5
  1-D Lookup Table : Lookup_n-D  NumberOfTableDimensions=1  BreakpointsForDimension1=SOD  Table=VOLT  InternalRulePriority=Speed  RndMeth=Simplest  InputSameDT=on
  Constant : Constant
  Gain : Gain  Gain=1.0985
  Gain1 : Gain  Gain=0.01
  MATLAB Function : MATLAB Function  TreatAsAtomicUnit=on
  Sum : Sum  Inputs=|-+
  To Workspace : ToWorkspace  VariableName=Umax  SaveFormat=Timeseries  SampleTime=-1
  To Workspace1 : ToWorkspace  Commented=on  VariableName=Ids_max  SampleTime=-1
  To Workspace2 : ToWorkspace  Commented=on  VariableName=regenmode  SampleTime=-1
  To Workspace4 : ToWorkspace  Commented=on  VariableName=Ich_max  SampleTime=-1
  To Workspace5 : ToWorkspace  Commented=on  VariableName=is_limited_complex  SampleTime=-1
  "id, ref2" : Constant  Value=Ich
  "id, ref3" : Constant  Value=vPart
  "id, ref4" : Constant  Value=soclim
  "id, ref6" : Constant  Value=aPart
  "id, ref8" : Constant  Value=Ids
  make decel. value positive : Gain  Gain=-1
  is_limited : Outport
  BrakeTrue : Outport  Port=2
  wires:
  MATLAB Function/1(is_limited) -> is_limited/1, To Workspace5/1
  isref/1 -> MATLAB Function/1(isref)
  "id, ref2"/1 -> MATLAB Function/2(Ich_m)
  "id, ref4"/1 -> MATLAB Function/4(soclim)
  "id, ref3"/1 -> MATLAB Function/6(vlimPartial)
  "id, ref6"/1 -> MATLAB Function/8(alimPartial)
  "id, ref8"/1 -> MATLAB Function/9(Ids_m)
  MATLAB Function/2(brakes) -> BrakeTrue/1
  soc/1 -> Gain1/1, MATLAB Function/3(soc)
  v/1 -> MATLAB Function/5(v)
  a/1 -> make decel. value positive/1
  make decel. value positive/1 -> MATLAB Function/7(a)
  Ubat/1 -> MATLAB Function/10(Ubat)
  Sum/1 -> 1-D Lookup Table/1
  Constant/1 -> Sum/2
  1-D Lookup Table/1 -> Gain/1
  Gain1/1 -> Sum/1
  MATLAB Function/5(mode) -> To Workspace2/1
  Gain/1 -> To Workspace/1, MATLAB Function/11(Umax)
  MATLAB Function/3(Ids_max) -> To Workspace1/1
  MATLAB Function/4(Ich_max) -> To Workspace4/1

== system ECB/ECB Model/Driver, Ctrl & Motor/TM saturation ==
  TM_ref : Inport
  wM : Inport  Port=2
  Divide2 : Product  Inputs=*/
  Gain : Gain  Gain=-1
  Maximum motor torque : Constant  Value=Tmax
  MinMax2 : MinMax  Inputs=2
  Peak power : Constant  Value=PmotPeak
  Saturation : Saturate  UpperLimit=inf  LowerLimit=0.01
  Saturation Dynamic1 : simulink/Discontinuities/Saturation Dynamic  OutMin=[]  OutMax=[]  OutDataTypeStr=Inherit: Same as second input  OutDataType=fixdt(1, 16)  OutScaling=2^-10  DoSatur=off
  To Workspace : ToWorkspace  VariableName=TMref  SampleTime=-1
      settings: Save2DSignal=2-D array (concatenate along first dimension)
  TMref_sat : Outport
  wires:
  Peak power/1 -> Divide2/1
  Maximum motor torque/1 -> MinMax2/2
  Divide2/1 -> MinMax2/1
  MinMax2/1 -> Gain/1, Saturation Dynamic1/1
  TM_ref/1 -> Saturation Dynamic1/2
  Saturation Dynamic1/1 -> To Workspace/1, TMref_sat/1
  wM/1 -> Saturation/1
  Gain/1 -> Saturation Dynamic1/3
  Saturation/1 -> Divide2/2

== system ECB/ECB Model/Energy Storage/Battery Dynamics ==
  i : Inport
  Delayed response : TransferFcn  Numerator=[R2]  Denominator=[(R2*C) 1]
  E : Sum  Inputs=+--
  Immediate response : Gain  Gain=R1
  Rate Limiter : RateLimiter  RisingSlewLimit=100  FallingSlewLimit=-100  SampleTimeMode=inherited
  SOD Calculation : Subsystem
  U : Outport
  SoC : Outport  Port=2
  wires:
  Immediate response/1 -> Rate Limiter/1
  E/1 -> U/1  "U"
  Delayed response/1 -> E/3
  SOD Calculation/2(SoC%) -> SoC/1
  i/1 -> Immediate response/1, Delayed response/1, SOD Calculation/1(i)
  SOD Calculation/1(Voc) -> E/1
  Rate Limiter/1 -> E/2

== system ECB/ECB Model/Energy Storage/Consumption ==
  i : Inport
  u : Inport  Port=2
  Integrator2 : Integrator
  Product : Product
  To Workspace3 : ToWorkspace  VariableName=kwh  SampleTime=-1
  ws->kwh1 : Gain  Gain=1/(3600*1000)
  wires:
  Product/1 -> Integrator2/1
  Integrator2/1 -> ws->kwh1/1
  i/1 -> Product/1
  u/1 -> Product/2
  ws->kwh1/1 -> To Workspace3/1

== system ECB/ECB Model/Energy Storage/Energy Recovery ==
  i : Inport
  Divide1 : Product  Inputs=/*
  Gain : Gain  Gain=-1
  Gain1 : Gain  Gain=100
  Integrator1 : Integrator  InitialCondition=1
  Integrator3 : Integrator
  Saturation : Saturate  UpperLimit=1000  LowerLimit=0
  Saturation1 : Saturate  UpperLimit=0  LowerLimit=-1000
  To Workspace3 : ToWorkspace  VariableName=reg  SampleTime=-1
  wires:
  Divide1/1 -> Gain1/1
  Saturation/1 -> Integrator1/1
  Gain/1 -> Integrator3/1
  Saturation1/1 -> Gain/1
  Integrator1/1 -> Divide1/1
  Integrator3/1 -> Divide1/2
  Gain1/1 -> To Workspace3/1
  i/1 -> Saturation/1, Saturation1/1

== system ECB/ECB Model/Mechanics/Elevation Calculation ==
  Sreal : Inport
  Grade : Inport  Port=2
  Add : Sum
  Clock : Clock
  Constant1 : Constant  Value=6.5
  Divide : Product  Inputs=*/
  Divide1 : Product  Inputs=**
  Integrator : Integrator
  Scope : Scope
  To Workspace3 : ToWorkspace  VariableName=Ele  SampleTime=-1
      settings: Save2DSignal=2-D array (concatenate along first dimension)
  Trigonometric Function2 : Trigonometry  Operator=tan  OutputSignalType=real
  wires:
  Add/1 -> Scope/1, To Workspace3/1
  Constant1/1 -> Add/1
  Trigonometric Function2/1 -> Integrator/1
  Clock/1 -> Divide/2
  Divide/1 -> Divide1/1
  Sreal/1 -> Divide/1
  Grade/1 -> Trigonometric Function2/1
  Integrator/1 -> Divide1/2
  Divide1/1 -> Add/2

== system ECB/ECB Model/Mechanics/Signal Builder ==
  Demux : Demux  Tag=STV Demux  Outputs=1
  FromWs : FromWorkspace  Tag=STV FromWs  VariableName=tuvar  SampleTime=0
      SigBuilderData=|
      | common.afterFinalStr = 'Extrapolate'
      | common.sampleTime = 0
      | dataSet.timeRange = [0 1548]
      | dataSet.name = 'GradeByLajunen'
      | sbobj.Groups.Name = 'GradeByLajunen'
      | sbobj.Groups.Signals.Name = 'vel'
      | sbobj.Groups.Signals.XData = [0 1 2 3 4 5 6 7 8 9 10 11 ... (1549 elements, 1x1549)]
      | sbobj.Groups.Signals.YData = [-0.00863189521262 -0.00863189521262 -0.00863189521262 -0.00863189521262 -0.00863189521262 -0.00863189521262 -0.00863189521262 -0.00863189521262 -0.00863189521262 -0.00863189521262 -0.00863189521262 -0.00863189521262 ... (1549 elements, 1x1549)]
      | sbobj.Groups.TimeRange = [0 1548]
  vel : Outport  Tag=STV Outport
  wires:
  Demux/1 -> vel/1
  FromWs/1 -> Demux/1

== system ECB/ECB Model/Driver, Ctrl & Motor/AC-motor/Electromagnetic Torque ==
  is : Inport
  psis : Inport  Port=2
  Complex to Real-Imag : ComplexToRealImag  Output=Imag
  Gain : Gain  Gain=(3/2)*p
  Math Function : Math  Operator=conj  SaturateOnIntegerOverflow=on
  Product : Product
  TM : Outport
  wires:
  Complex to Real-Imag/1 -> Gain/1
  Product/1 -> Complex to Real-Imag/1
  is/1 -> Product/1
  Gain/1 -> TM/1
  psis/1 -> Math Function/1
  Math Function/1 -> Product/2

== system ECB/ECB Model/Driver, Ctrl & Motor/AC-motor/Flux Equations ==
  psis : Inport
  Add : Sum  Inputs=+-
  Constant : Constant  Value=flux
  Gain2 : Gain  Gain=1/Ls
  IC : InitialCondition  Value=0
  Rate Limiter : RateLimiter  SampleTimeMode=inherited
  Scope : Scope
  is : Outport
  wires:
  Constant/1 -> IC/1
  psis/1 -> Add/1
  Add/1 -> Gain2/1
  Gain2/1 -> is/1
  IC/1 -> Rate Limiter/1
  Rate Limiter/1 -> Scope/1, Add/2
